simulink model "Sim"  (R2023b)
settings: Solver=ode5  StartTime=0.0  StopTime=time.value  RelTol=1e-3
undefined symbols (not defined in the file): chi2inv, clock, IMU, R_sensor2body
libraries: nav_lib x4, dyn_lib x2, simulink x1
settings Model: DataDictionary=SimulationDict.sldd  SimulationMode=accelerator  Creator=brent  LastModifiedBy=brent

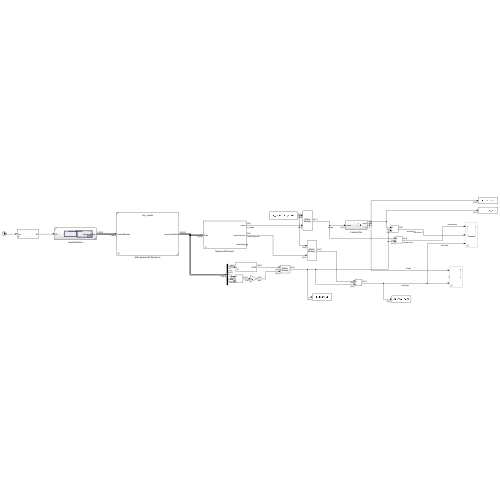
[thumbnail: Simulink's stored preview of the top-level diagram]
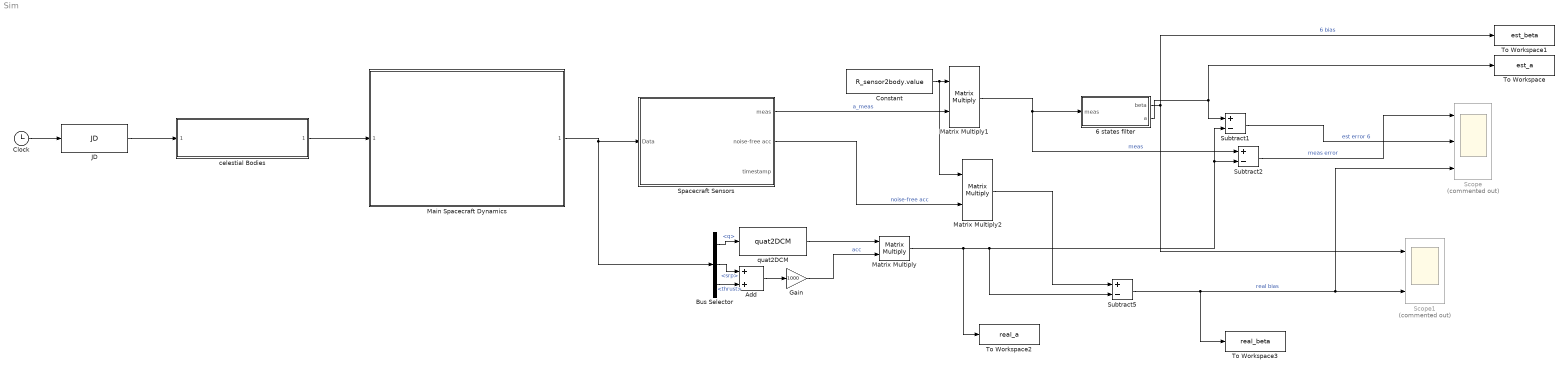
== system Sim ==
  6 states filter : Subsystem
  Add : Sum
  Bus Selector : BusSelector  OutputSignals=q,a.srp,a.thrust
  Clock : Clock
  Constant : Constant  Value=R_sensor2body.value
  Gain : Gain  Gain=1000
  JD : dyn_lib/JD  year=Environment.Date.year  month=Environment.Date.month  day=Environment.Date.day  hour=Environment.Date.hour  min=Environment.Date.min  sec=Environment.Date.sec
      settings: SourceProductName=Dynamics library
  Main Spacecraft Dynamics : Subsystem  ReferencedSubsystem=dyn_model  Environment=Environment  Spacecraft=MainSpacecraft  sc_type="\"main\""
  Matrix Multiply : Product  Multiplication=Matrix(*)
  Matrix Multiply1 : Product  Multiplication=Matrix(*)
  Matrix Multiply2 : Product  Multiplication=Matrix(*)
  Scope : Scope  Commented=on  NumInputPorts=3
  Scope1 : Scope  Commented=on  NumInputPorts=3
  Spacecraft Sensors : Subsystem
      mask DialogControl DescGroupVar Prompt: Main spacecraft sensors
  Subtract1 : Sum  Inputs=+-
  Subtract2 : Sum  Inputs=+-
  Subtract5 : Sum  Inputs=+-
  To Workspace : ToWorkspace  VariableName=est_a  SaveFormat=Timeseries  SampleTime=-1
  To Workspace1 : ToWorkspace  VariableName=est_beta  SaveFormat=Timeseries  SampleTime=-1
  To Workspace2 : ToWorkspace  VariableName=real_a  SampleTime=-1
  To Workspace3 : ToWorkspace  VariableName=real_beta  SampleTime=-1
  celestial Bodies : Subsystem  ReferencedSubsystem=celestialBodies
      settings: PermitHierarchicalResolution=None
  quat2DCM : dyn_lib/quat2DCM
      settings: SourceProductName=Dynamics library
  wires:
  celestial Bodies/1 -> Main Spacecraft Dynamics/1
  Clock/1 -> JD/1
  JD/1 -> celestial Bodies/1
  Main Spacecraft Dynamics/1 -> Bus Selector/1, Spacecraft Sensors/1(Data)
  Spacecraft Sensors/1(meas) -> Matrix Multiply1/2  "a_meas"
  Bus Selector/2 -> Add/1  "<srp>"
  Bus Selector/3 -> Add/2  "<thrust>"
  Add/1 -> Gain/1
  6 states filter/1(beta) -> Scope1/1, To Workspace1/1  "6 bias"
  Subtract1/1 -> Scope/2  "est error 6"
  Gain/1 -> Matrix Multiply/2  "acc"
  Bus Selector/1 -> quat2DCM/1  "<q>"
  Matrix Multiply/1 -> Subtract1/2, Subtract2/2, Subtract5/2, To Workspace2/1
  Subtract2/1 -> Scope/1  "meas error"
  quat2DCM/1 -> Matrix Multiply/1
  Constant/1 -> Matrix Multiply2/1, Matrix Multiply1/1
  Matrix Multiply1/1 -> Subtract2/1, 6 states filter/1(meas)  "meas"
  Subtract5/1 -> To Workspace3/1, Scope/3, Scope1/3  "real bias"
  Matrix Multiply2/1 -> Subtract5/1
  Spacecraft Sensors/2(noise-free acc) -> Matrix Multiply2/2  "noise-free acc"
  6 states filter/2(a) -> Subtract1/1, To Workspace/1

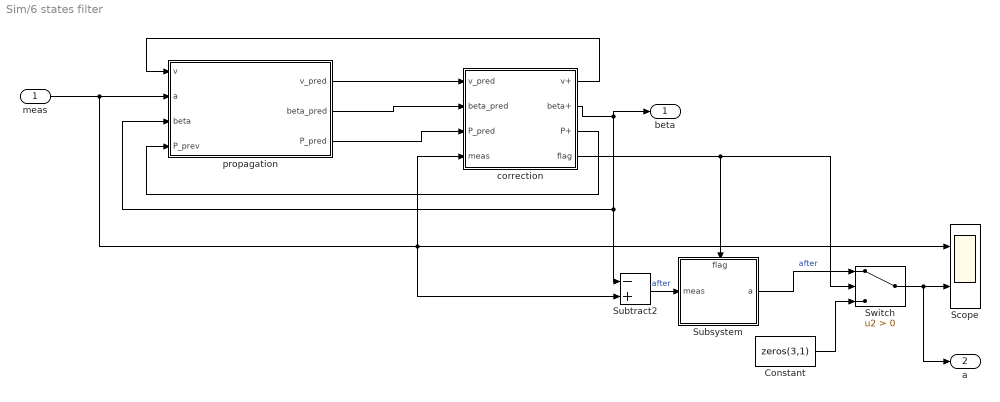
== system Sim/6 states filter ==
  meas : Inport
  Constant : Constant  Value=zeros(3,1)  VectorParams1D=off
  Scope : Scope  NumInputPorts=2
  Subsystem : Subsystem
      settings: PortSchema="{\"entries\":[{\"content\":{\"sides\":[{\"content\":{\"connectorIds\":[\"In1\"]},\"type\":\"ConnectorPlacement.EquallySpacedRectSide\",\"uuid\":\"04984c6d-68bb-4868-b555-561b55ad66cf\"},{\"content\":{\"connectorIds\":[\"Out1\"],\"side\":\"RIGHT\"},\"type\":\"ConnectorPlacement.EquallySpacedRectSide\",\"uuid\":\"a81d3184-9e13-42c8-a176-83bd8c1c8126\"},{\"content\":{\"connectorIds\":[\"In2\"],\"side\":\"TOP\"},\"type\":\"ConnectorPlacement.EquallySpacedRectSide\",\"uuid\":\"95046c64-69a7-4e42-aa3a-b7d167259f83\"}]},\"type\":\"ConnectorPlacement.EquallySpacedConnector\",\"uuid\":\"a38104d1-1e85-4f2e-aa1d-28155c2663e4\"}],\"packageUris\":[\"http://schema.mathworks.com/mf0/Connector/R2020b\"],\"version\":\"1.0\"}"
  Subtract2 : Sum  Inputs=-+
  Switch : Switch  Criteria=u2 > Threshold  SaturateOnIntegerOverflow=off  InputSameDT=off
  correction : Subsystem
  propagation : Subsystem  mask{dt=IMU.accelerometer.sampleTime.value}
      mask prompts: dt "sample time"
      mask DialogControl DescGroupVar Prompt: Propagation Step
  beta : Outport
  a : Outport  Port=2
  wires:
  correction/2(beta+) -> beta/1, Subtract2/1, propagation/3(beta)
  correction/3(P+) -> propagation/4(P_prev)
  propagation/2(beta_pred) -> correction/2(beta_pred)
  propagation/3(P_pred) -> correction/3(P_pred)
  propagation/1(v_pred) -> correction/1(v_pred)
  correction/1(v+) -> propagation/1(v)
  correction/4(flag) -> Subsystem/2(flag), Switch/2
  Switch/1 -> a/1, Scope/2
  Constant/1 -> Switch/3
  Subsystem/1(a) -> Switch/1  "after"
  Subtract2/1 -> Subsystem/1(meas)  "after"
  meas/1 -> correction/4(meas), Subtract2/2, Scope/1, propagation/2(a)

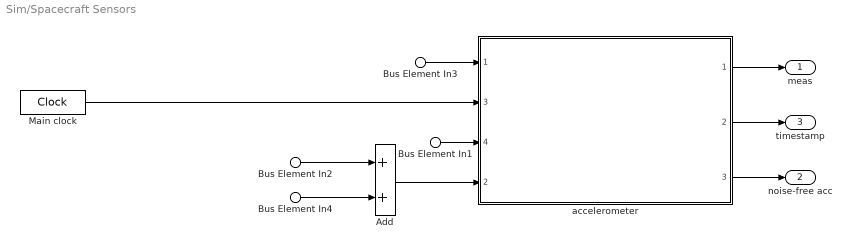
== system Sim/Spacecraft Sensors ==
  Bus Element In3 : Inport  PortName=Data  Element=w
  Bus Element In1 : Inport  PortName=Data  Element=q
  Bus Element In2 : Inport  PortName=Data  Element=a.srp
  Bus Element In4 : Inport  PortName=Data  Element=a.thrust
  Add : Sum
  Main clock : DigitalClock  SampleTime=clock.sampleTime.value
  accelerometer : Subsystem  TreatAsAtomicUnit=on  SystemSampleTime=IMU.accelerometer.sampleTime.value  ReferencedSubsystem=accelerometer
      settings: PortSchema="{\"entries\":[{\"content\":{\"sides\":[{\"content\":{\"connectorIds\":[\"In1\",\"In3\",\"In4\",\"In2\"]},\"type\":\"ConnectorPlacement.EquallySpacedRectSide\",\"uuid\":\"f690aca1-0f02-47fc-8596-4493e25f285c\"},{\"content\":{\"connectorIds\":[\"Out1\",\"Out2\",\"Out3\"],\"side\":\"RIGHT\"},\"type\":\"ConnectorPlacement.EquallySpacedRectSide\",\"uuid\":\"ecd25334-8389-4aa4-af3e-65bbeaac2b4b\"},{\"content\":{\"side\":\"TOP\"},\"type\":\"ConnectorPlacement.EquallySpacedRectSide\",\"uuid\":\"886a7907-fe4b-4c0c-bdd8-227e17cf6450\"}]},\"type\":\"ConnectorPlacement.EquallySpacedConnector\",\"uuid\":\"5845c284-1d3d-44f6-9189-c640147e7586\"}],\"packageUris\":[\"http://schema.mathworks.com/mf0/Connector/R2020b\"],\"version\":\"1.0\"}"
  meas : Outport
  noise-free acc : Outport  Port=2
  timestamp : Outport  Port=3
  wires:
  Bus Element In3/1 -> accelerometer/1
  Bus Element In1/1 -> accelerometer/4
  Main clock/1 -> accelerometer/3
  Bus Element In2/1 -> Add/1
  Bus Element In4/1 -> Add/2
  accelerometer/2 -> timestamp/1
  accelerometer/1 -> meas/1
  accelerometer/3 -> noise-free acc/1
  Add/1 -> accelerometer/2

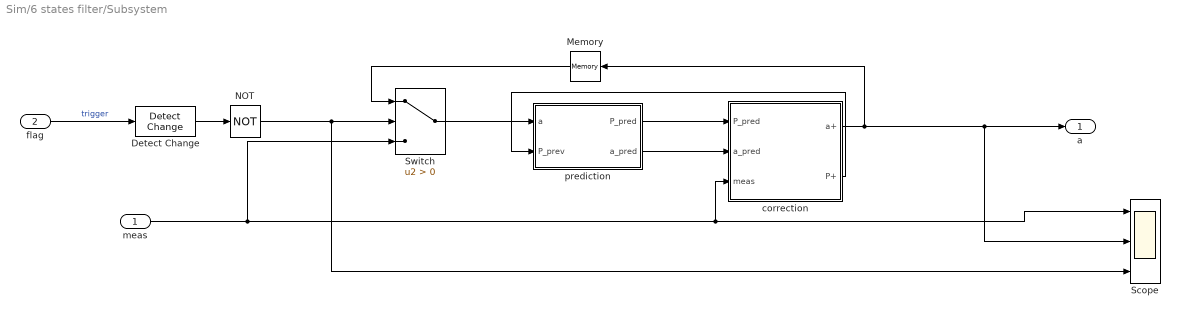
== system Sim/6 states filter/Subsystem ==
  meas : Inport
  flag : Inport  Port=2
  Detect Change : simulink/Logic and Bit Operations/Detect Change  vinit=0  OutDataTypeStr=boolean
  Memory : Memory
  NOT : Logic  Operator=NOT  IconShape=distinctive  AllPortsSameDT=off  OutDataTypeStr=boolean
  Scope : Scope  NumInputPorts=3
  Switch : Switch  Criteria=u2 > Threshold  SaturateOnIntegerOverflow=off  InputSameDT=off
  correction : Subsystem
  prediction : Subsystem
  a : Outport
  wires:
  prediction/1(P_pred) -> correction/1(P_pred)
  prediction/2(a_pred) -> correction/2(a_pred)
  correction/2(P+) -> prediction/2(P_prev)
  Switch/1 -> prediction/1(a)
  correction/1(a+) -> Memory/1, Scope/2, a/1
  flag/1 -> Detect Change/1  "trigger"
  meas/1 -> Scope/1, correction/3(meas), Switch/3
  Memory/1 -> Switch/1
  NOT/1 -> Scope/3, Switch/2
  Detect Change/1 -> NOT/1

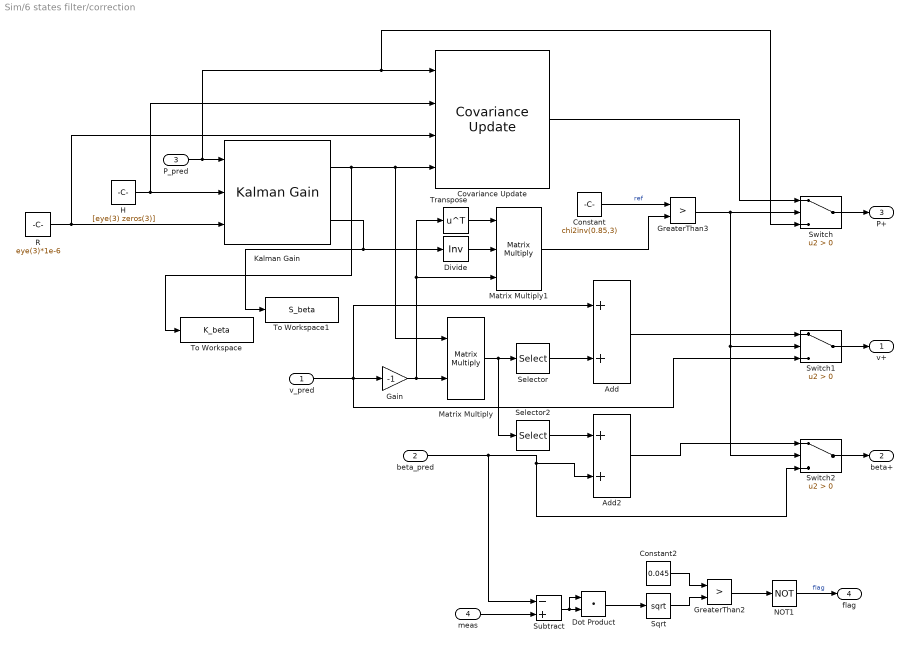
== system Sim/6 states filter/correction ==
  v_pred : Inport
  beta_pred : Inport  Port=2
  P_pred : Inport  Port=3
  meas : Inport  Port=4
  Add : Sum
  Add2 : Sum
  Constant : Constant  Value=chi2inv(0.85,3)
  Constant2 : Constant  Value=0.045
  Covariance Update : nav_lib/Covariance Update
      settings: SourceProductName=Navigation library
  Divide : Product  Inputs=/  Multiplication=Matrix(*)
  Dot Product : DotProduct  OutDataTypeStr=Inherit: Inherit via internal rule
  Gain : Gain  Gain=-1
  GreaterThan2 : RelationalOperator  Operator=>  OutDataTypeStr=boolean  RndMeth=Simplest  InputSameDT=off
  GreaterThan3 : RelationalOperator  Operator=>  OutDataTypeStr=boolean  RndMeth=Simplest  InputSameDT=off
  H : Constant  Value=[eye(3) zeros(3)]
  Kalman Gain : nav_lib/Kalman Gain
      settings: SourceProductName=Navigation library
  Matrix Multiply : Product  Multiplication=Matrix(*)
  Matrix Multiply1 : Product  Inputs=3  Multiplication=Matrix(*)
  NOT1 : Logic  Operator=NOT  IconShape=distinctive  AllPortsSameDT=off  OutDataTypeStr=boolean
  R : Constant  Value=eye(3)*1e-6
  Selector : Selector  NumberOfDimensions=2  InputPortWidth=3  IndexOptions=Index vector (dialog),Select all  Indices=1:3,1  OutputSizes=1,1
  Selector2 : Selector  NumberOfDimensions=2  InputPortWidth=3  IndexOptions=Index vector (dialog),Select all  Indices=4:6,1  OutputSizes=1,1
  Sqrt : Sqrt
  Subtract : Sum  Inputs=-+
  Switch : Switch  Criteria=u2 > Threshold  SaturateOnIntegerOverflow=off  InputSameDT=off
  Switch1 : Switch  Criteria=u2 > Threshold  SaturateOnIntegerOverflow=off  InputSameDT=off
  Switch2 : Switch  Criteria=u2 > Threshold  SaturateOnIntegerOverflow=off  InputSameDT=off
  To Workspace : ToWorkspace  VariableName=K_beta  SaveFormat=Timeseries  SampleTime=-1
  To Workspace1 : ToWorkspace  VariableName=S_beta  SaveFormat=Timeseries  SampleTime=-1
  Transpose : Math  Operator=transpose
  v+ : Outport
  beta+ : Outport  Port=2
  P+ : Outport  Port=3
  flag : Outport  Port=4
  wires:
  beta_pred/1 -> Subtract/1, Switch2/3, Add2/2
  Selector2/1 -> Add2/1
  Selector/1 -> Add/2
  Matrix Multiply/1 -> Selector/1, Selector2/1
  Gain/1 -> Matrix Multiply1/3, Transpose/1, Matrix Multiply/2
  v_pred/1 -> Switch1/3, Add/1, Gain/1
  H/1 -> Kalman Gain/2, Covariance Update/2
  P_pred/1 -> Kalman Gain/1, Switch/3, Covariance Update/1
  R/1 -> Kalman Gain/3, Covariance Update/3
  Kalman Gain/1 -> To Workspace/1, Covariance Update/4, Matrix Multiply/1
  Transpose/1 -> Matrix Multiply1/1
  Divide/1 -> Matrix Multiply1/2
  Constant/1 -> GreaterThan3/1  "ref"
  Matrix Multiply1/1 -> GreaterThan3/2
  GreaterThan3/1 -> Switch/2, Switch1/2, Switch2/2
  Switch/1 -> P+/1
  Covariance Update/1 -> Switch/1
  Add/1 -> Switch1/1
  Switch1/1 -> v+/1
  Switch2/1 -> beta+/1
  Add2/1 -> Switch2/1
  Kalman Gain/2 -> Divide/1, To Workspace1/1
  Sqrt/1 -> GreaterThan2/2
  Constant2/1 -> GreaterThan2/1
  GreaterThan2/1 -> NOT1/1
  Dot Product/1 -> Sqrt/1
  NOT1/1 -> flag/1  "flag"
  Subtract/1 -> Dot Product/1, Dot Product/2
  meas/1 -> Subtract/2

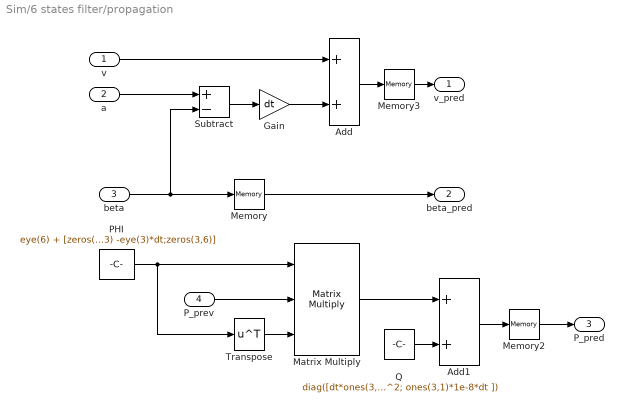
== system Sim/6 states filter/propagation ==
  v : Inport
  a : Inport  Port=2
  beta : Inport  Port=3
  P_prev : Inport  Port=4
  Add : Sum
  Add1 : Sum
  Gain : Gain  Gain=dt
  Matrix Multiply : Product  Inputs=3  Multiplication=Matrix(*)
  Memory : Memory  InitialCondition=zeros(3,1)
  Memory2 : Memory  InitialCondition=eye(6)*1e-4
  Memory3 : Memory  InitialCondition=zeros(3,1)
  PHI : Constant  Value=eye(6) + [zeros(3) -eye(3)*dt;zeros(3,6)]
  Q : Constant  Value=diag([dt*ones(3,1)*IMU.accelerometer.N.value^2-dt*ones(3,1)*IMU.accelerometer.K.value^2; ones(3,1)*1e-8*dt ])
  Subtract : Sum  Inputs=+-
  Transpose : Math  Operator=transpose
  v_pred : Outport
  beta_pred : Outport  Port=2
  P_pred : Outport  Port=3
  wires:
  Add1/1 -> Memory2/1
  Matrix Multiply/1 -> Add1/1
  Q/1 -> Add1/2
  P_prev/1 -> Matrix Multiply/2
  Transpose/1 -> Matrix Multiply/3
  PHI/1 -> Matrix Multiply/1, Transpose/1
  Add/1 -> Memory3/1
  v/1 -> Add/1
  Gain/1 -> Add/2
  Subtract/1 -> Gain/1
  a/1 -> Subtract/1
  beta/1 -> Memory/1, Subtract/2
  Memory/1 -> beta_pred/1
  Memory3/1 -> v_pred/1
  Memory2/1 -> P_pred/1

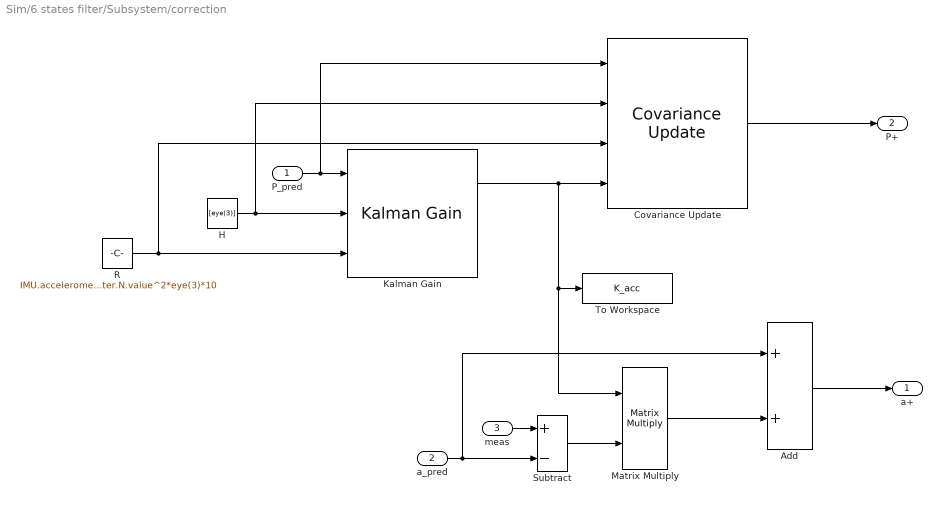
== system Sim/6 states filter/Subsystem/correction ==
  P_pred : Inport
  a_pred : Inport  Port=2
  meas : Inport  Port=3
  Add : Sum
  Covariance Update : nav_lib/Covariance Update
      settings: SourceProductName=Navigation library
  H : Constant  Value=[eye(3)]
  Kalman Gain : nav_lib/Kalman Gain
      settings: SourceProductName=Navigation library
  Matrix Multiply : Product  Multiplication=Matrix(*)
  R : Constant  Value=IMU.accelerometer.N.value^2*eye(3)*10
  Subtract : Sum  Inputs=+-
  To Workspace : ToWorkspace  VariableName=K_acc  SaveFormat=Timeseries  SampleTime=-1
  a+ : Outport
  P+ : Outport  Port=2
  wires:
  Kalman Gain/1 -> Matrix Multiply/1, To Workspace/1, Covariance Update/4
  R/1 -> Covariance Update/3, Kalman Gain/3
  P_pred/1 -> Covariance Update/1, Kalman Gain/1
  H/1 -> Covariance Update/2, Kalman Gain/2
  a_pred/1 -> Add/1, Subtract/2
  Subtract/1 -> Matrix Multiply/2
  Matrix Multiply/1 -> Add/2
  meas/1 -> Subtract/1
  Add/1 -> a+/1
  Covariance Update/1 -> P+/1

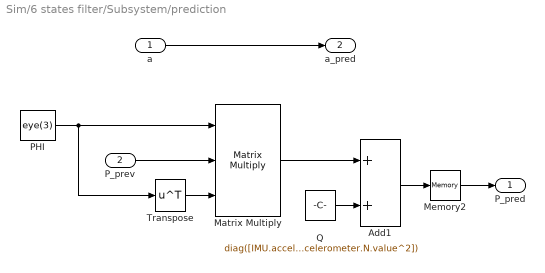
== system Sim/6 states filter/Subsystem/prediction ==
  a : Inport
  P_prev : Inport  Port=2
  Add1 : Sum
  Matrix Multiply : Product  Inputs=3  Multiplication=Matrix(*)
  Memory2 : Memory  InitialCondition=eye(3)*IMU.accelerometer.N.value^2
  PHI : Constant  Value=eye(3)
  Q : Constant  Value=diag([IMU.accelerometer.sampleTime.value*ones(3,1)*IMU.accelerometer.N.value^2])
  Transpose : Math  Operator=transpose
  P_pred : Outport
  a_pred : Outport  Port=2
  wires:
  Transpose/1 -> Matrix Multiply/3
  Add1/1 -> Memory2/1
  P_prev/1 -> Matrix Multiply/2
  PHI/1 -> Matrix Multiply/1, Transpose/1
  Matrix Multiply/1 -> Add1/1
  Memory2/1 -> P_pred/1
  Q/1 -> Add1/2
  a/1 -> a_pred/1
